simulink library "my_library"  (R2014a)
settings: Solver=ode45  StartTime=0.0  StopTime=10.0  RelTol=1e-3
values from neighbouring files (symbols this model uses):
  D = D~=0    [diffTimeSeries.m]    (also in scenario_visualizer_gui.m = D+diffTimeSeries(scenario.failure.communication.packet_recei)
undefined symbols (not defined in the file or in its folder): cmd_delay, decStep, decStepMax, incStep
libraries: my_library x27, simulink x1
settings Model: Creator=jean  LastModifiedBy=jean

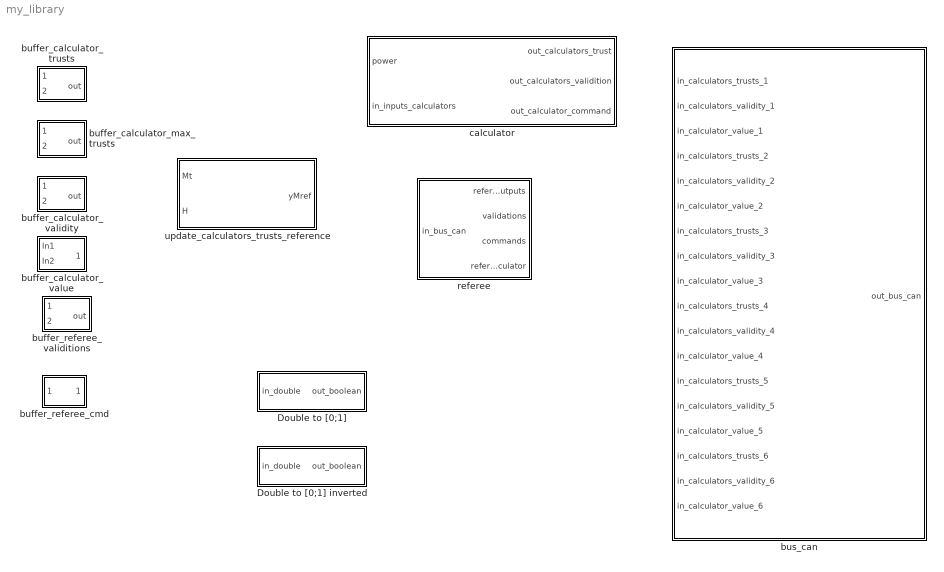
== system my_library ==
  Double to [0;1] : Subsystem
  Double to [0;1] inverted : Subsystem
  buffer_calculator_max_trusts : Subsystem
  buffer_calculator_trusts : Subsystem
  buffer_calculator_validity : Subsystem
  buffer_calculator_value : Subsystem
  buffer_referee_cmd : Subsystem
  buffer_referee_validitions : Subsystem
  bus_can : Subsystem
      mask Display: image('images/network_grid.jpg');
  calculator : Subsystem  mask{id=0}
      mask prompts: id "Component ID"
      mask init:
      | id>=1
      mask Display: image('images/stm32f4_discovery.jpg');
  referee : Subsystem  mask{cmd_delay=4}
      mask prompts: cmd_delay "Command delay"
      mask Display: image('images/984838-brain.jpg');
  update_calculators_trusts_reference : MATLAB Function  TreatAsAtomicUnit=on

== system my_library/Double to [0;1] ==
  in_double : Inport
  Constant : Constant  Value=0
  Constant1 : Constant
  Switch : Switch  Threshold=0.5
  out_boolean : Outport
  wires:
  Constant/1 -> Switch/3
  Constant1/1 -> Switch/1
  Switch/1 -> out_boolean/1
  in_double/1 -> Switch/2

== system my_library/Double to [0;1] inverted ==
  in_double : Inport
  Constant : Constant
  Constant1 : Constant  Value=0
  Switch : Switch  Threshold=0.5
  out_boolean : Outport
  wires:
  in_double/1 -> Switch/2
  Switch/1 -> out_boolean/1
  Constant1/1 -> Switch/1
  Constant/1 -> Switch/3

== system my_library/buffer_calculator_max_trusts ==
  input : Inport
  reset : Inport  Port=2
  Delay18 : Delay  DelayLength=1  InitialCondition=ones(1,9,'double')  ExternalReset=Level hold
      settings: InputPortMap=u0,r5
  Reshape12 : Reshape  OutputDimensionality=Row vector (2-D)  OutputDimensions=[6,6]
  out : Outport
  wires:
  Delay18/1 -> Reshape12/1
  input/1 -> Delay18/1
  Reshape12/1 -> out/1
  reset/1 -> Delay18/2

== system my_library/buffer_calculator_trusts ==
  input : Inport
  reset : Inport  Port=2
  Reshape : Reshape  OutputDimensionality=Row vector (2-D)  OutputDimensions=[6,6]
  calculator_buffer_trusts : Delay  DelayLength=1  InitialCondition=ones(1,6,'double')  ExternalReset=Level hold
      settings: InputPortMap=u0,r5
  out : Outport
  wires:
  reset/1 -> calculator_buffer_trusts/2
  calculator_buffer_trusts/1 -> Reshape/1
  input/1 -> calculator_buffer_trusts/1
  Reshape/1 -> out/1

== system my_library/buffer_calculator_validity ==
  input : Inport
  reset : Inport  Port=2
  Delay6 : Delay  DelayLength=1  InitialCondition=cast(zeros(1,6),'int8')  ExternalReset=Level hold
      settings: InputPortMap=u0,r5
  Reshape6 : Reshape  OutputDimensionality=Row vector (2-D)  OutputDimensions=[6,6]
  out : Outport
  wires:
  input/1 -> Delay6/1
  Reshape6/1 -> out/1
  Delay6/1 -> Reshape6/1
  reset/1 -> Delay6/2

== system my_library/buffer_calculator_value ==
  In1 : Inport
  In2 : Inport  Port=2
  Delay : Delay  DelayLength=1  ExternalReset=Level hold
      settings: InputPortMap=u0,r5
  Out1 : Outport
  wires:
  Delay/1 -> Out1/1
  In1/1 -> Delay/1
  In2/1 -> Delay/2

== system my_library/buffer_referee_cmd ==
  In1 : Inport
  calculators_validity_6 : Delay  DelayLength=cmd_delay  InitialCondition=0
  Out1 : Outport
  wires:
  In1/1 -> calculators_validity_6/1
  calculators_validity_6/1 -> Out1/1

== system my_library/buffer_referee_validitions ==
  input : Inport
  reset : Inport  Port=2
  Delay6 : Delay  DelayLength=cmd_delay-1  InitialCondition=0  ExternalReset=Level hold
      settings: InputPortMap=u0,r5
  Reshape6 : Reshape  OutputDimensionality=Row vector (2-D)  OutputDimensions=[6,6]
  out : Outport
  wires:
  input/1 -> Delay6/1
  Reshape6/1 -> out/1
  Delay6/1 -> Reshape6/1
  reset/1 -> Delay6/2

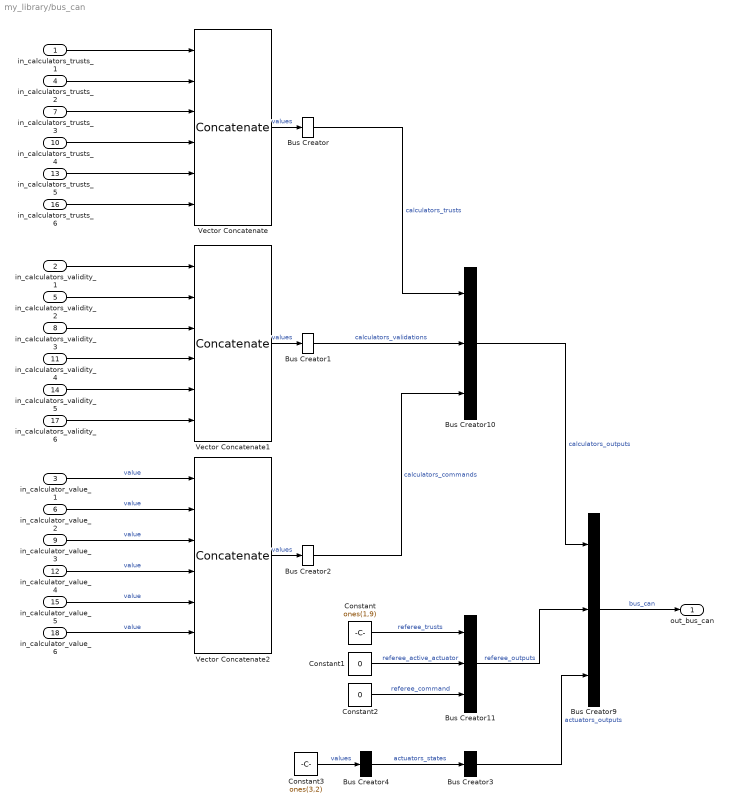
== system my_library/bus_can ==
  in_calculators_trusts_1 : Inport
  in_calculators_validity_1 : Inport  Port=2
  in_calculator_value_1 : Inport  Port=3  OutDataTypeStr=double  PortDimensions=1
  in_calculators_trusts_2 : Inport  Port=4
  in_calculators_validity_2 : Inport  Port=5
  in_calculator_value_2 : Inport  Port=6  OutDataTypeStr=double  PortDimensions=1
  in_calculators_trusts_3 : Inport  Port=7
  in_calculators_validity_3 : Inport  Port=8
  in_calculator_value_3 : Inport  Port=9  OutDataTypeStr=double  PortDimensions=1
  in_calculators_trusts_4 : Inport  Port=10
  in_calculators_validity_4 : Inport  Port=11
  in_calculator_value_4 : Inport  Port=12  OutDataTypeStr=double  PortDimensions=1
  in_calculators_trusts_5 : Inport  Port=13
  in_calculators_validity_5 : Inport  Port=14
  in_calculator_value_5 : Inport  Port=15  OutDataTypeStr=double  PortDimensions=1
  in_calculators_trusts_6 : Inport  Port=16
  in_calculators_validity_6 : Inport  Port=17
  in_calculator_value_6 : Inport  Port=18  OutDataTypeStr=double  PortDimensions=1
  Bus Creator : BusCreator  Inputs=1  OutDataTypeStr=Bus: bus_calculators_trusts
  Bus Creator1 : BusCreator  Inputs=1  OutDataTypeStr=Bus: bus_calculators_validations
  Bus Creator10 : BusCreator  Inputs=3  OutDataTypeStr=Bus: bus_calculators_outputs
  Bus Creator11 : BusCreator  Inputs=3  OutDataTypeStr=Bus: bus_referee_outputs
  Bus Creator2 : BusCreator  Inputs=1  OutDataTypeStr=Bus: bus_calculators_commands
  Bus Creator3 : BusCreator  Inputs=1  OutDataTypeStr=Bus: bus_actuators_outputs
  Bus Creator4 : BusCreator  Inputs=1  OutDataTypeStr=Bus: bus_actuators_states
  Bus Creator9 : BusCreator  Inputs=3  OutDataTypeStr=Bus: bus_can
  Constant : Constant  Value=ones(1,9)
  Constant1 : Constant  Value=0
  Constant2 : Constant  Value=0
  Constant3 : Constant  Value=ones(3,2)  VectorParams1D=off
  Vector Concatenate : Concatenate  NumInputs=6  Mode=Multidimensional array
  Vector Concatenate1 : Concatenate  NumInputs=6  Mode=Multidimensional array
  Vector Concatenate2 : Concatenate  NumInputs=6  Mode=Multidimensional array
  out_bus_can : Outport  OutDataTypeStr=Bus: bus_can
  wires:
  Vector Concatenate/1 -> Bus Creator/1  "values"
  Vector Concatenate1/1 -> Bus Creator1/1  "values"
  Vector Concatenate2/1 -> Bus Creator2/1  "values"
  in_calculators_trusts_4/1 -> Vector Concatenate/4
  in_calculators_trusts_1/1 -> Vector Concatenate/1
  in_calculators_trusts_5/1 -> Vector Concatenate/5
  in_calculators_trusts_3/1 -> Vector Concatenate/3
  in_calculators_trusts_2/1 -> Vector Concatenate/2
  in_calculators_trusts_6/1 -> Vector Concatenate/6
  in_calculators_validity_4/1 -> Vector Concatenate1/4
  in_calculators_validity_1/1 -> Vector Concatenate1/1
  in_calculators_validity_5/1 -> Vector Concatenate1/5
  in_calculators_validity_6/1 -> Vector Concatenate1/6
  in_calculators_validity_3/1 -> Vector Concatenate1/3
  in_calculators_validity_2/1 -> Vector Concatenate1/2
  in_calculator_value_6/1 -> Vector Concatenate2/6  "value"
  in_calculator_value_1/1 -> Vector Concatenate2/1  "value"
  in_calculator_value_3/1 -> Vector Concatenate2/3  "value"
  in_calculator_value_2/1 -> Vector Concatenate2/2  "value"
  in_calculator_value_4/1 -> Vector Concatenate2/4  "value"
  in_calculator_value_5/1 -> Vector Concatenate2/5  "value"
  Bus Creator9/1 -> out_bus_can/1  "bus_can"
  Bus Creator10/1 -> Bus Creator9/1  "calculators_outputs"
  Bus Creator/1 -> Bus Creator10/1  "calculators_trusts"
  Bus Creator1/1 -> Bus Creator10/2  "calculators_validations"
  Bus Creator2/1 -> Bus Creator10/3  "calculators_commands"
  Bus Creator11/1 -> Bus Creator9/2  "referee_outputs"
  Bus Creator3/1 -> Bus Creator9/3  "actuators_outputs"
  Constant/1 -> Bus Creator11/1  "referee_trusts"
  Constant1/1 -> Bus Creator11/2  "referee_active_actuator"
  Constant2/1 -> Bus Creator11/3  "referee_command"
  Bus Creator4/1 -> Bus Creator3/1  "actuators_states"
  Constant3/1 -> Bus Creator4/1  "values"

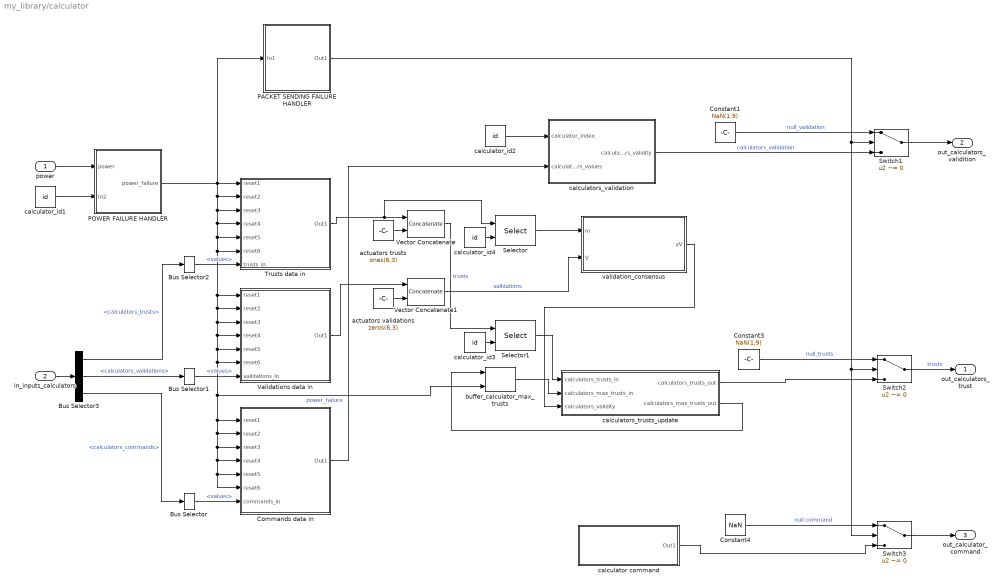
== system my_library/calculator ==
  power : Inport  OutMin=0  OutMax=1  PortDimensions=1
  in_inputs_calculators : Inport  Port=2  OutDataTypeStr=Bus: bus_can
  Bus Selector : BusSelector  OutputSignals=values
  Bus Selector1 : BusSelector  OutputSignals=values
  Bus Selector2 : BusSelector  OutputSignals=values
  Bus Selector3 : BusSelector  OutputSignals=calculators_outputs.calculators_trusts,calculators_outputs.calculators_validations,calculators_outputs.calculators_commands
  Commands data in : Subsystem
  Constant1 : Constant  Value=NaN(1,9)  VectorParams1D=off
  Constant3 : Constant  Value=NaN(1,9)  VectorParams1D=off
  Constant4 : Constant  Value=NaN  VectorParams1D=off
  PACKET SENDING FAILURE HANDLER : Subsystem
  POWER FAILURE HANDLER : Subsystem
      mask Display: image('images/electricity_failure.jpg');
  Selector : Selector  NumberOfDimensions=2  InputPortWidth=6  IndexOptions=Index vector (port),Select all  Indices=[1 3],1  OutputSizes=1,1
  Selector1 : Selector  NumberOfDimensions=2  InputPortWidth=6  IndexOptions=Index vector (port),Select all  Indices=[1 3],1  OutputSizes=1,1
  Switch1 : Switch  Criteria=u2 ~= 0
  Switch2 : Switch  Criteria=u2 ~= 0
  Switch3 : Switch  Criteria=u2 ~= 0
  Trusts data in : Subsystem
  Validations data in : Subsystem
  Vector Concatenate : Concatenate  Mode=Multidimensional array  ConcatenateDimension=2
  Vector Concatenate1 : Concatenate  Mode=Multidimensional array  ConcatenateDimension=2
  actuators trusts : Constant  Value=ones(6,3)  VectorParams1D=off
  actuators validations : Constant  Value=zeros(6,3)  VectorParams1D=off
  buffer_calculator_max_trusts : my_library/buffer_calculator_max_trusts
  calculator command : Subsystem
  calculator_id{1..4} (4 alike) : Constant  Value=id  OutDataTypeStr=uint8
  calculators_trusts_update : Subsystem
  calculators_validation : Subsystem
  validation_consensus : MATLAB Function  TreatAsAtomicUnit=on
  out_calculators_trust : Outport
  out_calculators_validition : Outport  Port=2
  out_calculator_command : Outport  Port=3  OutDataTypeStr=double  PortDimensions=1
  wires:
  calculator_id1/1 -> POWER FAILURE HANDLER/2(In2)
  in_inputs_calculators/1 -> Bus Selector3/1
  validation_consensus/1(yV) -> calculators_trusts_update/3(calculators_validity)
  calculators_trusts_update/1(calculators_trusts_out) -> Switch2/3
  Selector/1 -> validation_consensus/1(m)
  calculators_trusts_update/2(calculators_max_trusts_out) -> buffer_calculator_max_trusts/1
  buffer_calculator_max_trusts/1 -> calculators_trusts_update/2(calculators_max_trusts_in)
  Switch1/1 -> out_calculators_validition/1
  calculators_validation/1(calculators_validity) -> Switch1/3  "calculators_validation"
  Constant1/1 -> Switch1/1  "null_validation"
  Switch2/1 -> out_calculators_trust/1  "trusts"
  Constant3/1 -> Switch2/1  "null_trusts"
  Switch3/1 -> out_calculator_command/1
  Constant4/1 -> Switch3/1  "null command"
  POWER FAILURE HANDLER/1(power_failure) -> buffer_calculator_max_trusts/2, Commands data in/6(reset6), Commands data in/5(reset5), Commands data in/4(reset4), Commands data in/3(reset3), Commands data in/2(reset2), Commands data in/1(reset1), Validations data in/6(reset6), Validations data in/5(reset5), Validations data in/4(reset4), Validations data in/3(reset3), Validations data in/2(reset2), Validations data in/1(reset1), Trusts data in/6(reset6), Trusts data in/5(reset5), Trusts data in/4(reset4), Trusts data in/3(reset3), Trusts data in/2(reset2), PACKET SENDING FAILURE HANDLER/1(In1), Trusts data in/1(reset1)  "power_failure"
  power/1 -> POWER FAILURE HANDLER/1(power)
  Bus Selector3/1 -> Bus Selector2/1  "<calculators_trusts>"
  Trusts data in/1(Out1) -> Selector/1, Vector Concatenate/1
  Bus Selector3/2 -> Bus Selector1/1  "<calculators_validations>"
  Bus Selector/1 -> Commands data in/7(commands_in)  "<values>"
  Commands data in/1(Out1) -> calculators_validation/2(calculators_values)
  calculator_id2/1 -> calculators_validation/1(calculator_index)
  actuators trusts/1 -> Vector Concatenate/2
  calculator_id4/1 -> Selector/2
  actuators validations/1 -> Vector Concatenate1/2
  Validations data in/1(Out1) -> Vector Concatenate1/1
  Vector Concatenate1/1 -> validation_consensus/2(V)  "validations"
  calculator command/1(Out1) -> Switch3/3
  calculator_id3/1 -> Selector1/2
  Vector Concatenate/1 -> Selector1/1  "trusts"
  Selector1/1 -> calculators_trusts_update/1(calculators_trusts_in)
  Bus Selector3/3 -> Bus Selector/1  "<calculators_commands>"
  Bus Selector1/1 -> Validations data in/7(validations_in)  "<values>"
  Bus Selector2/1 -> Trusts data in/7(trusts_in)  "<values>"
  PACKET SENDING FAILURE HANDLER/1(Out1) -> Switch3/2, Switch2/2, Switch1/2

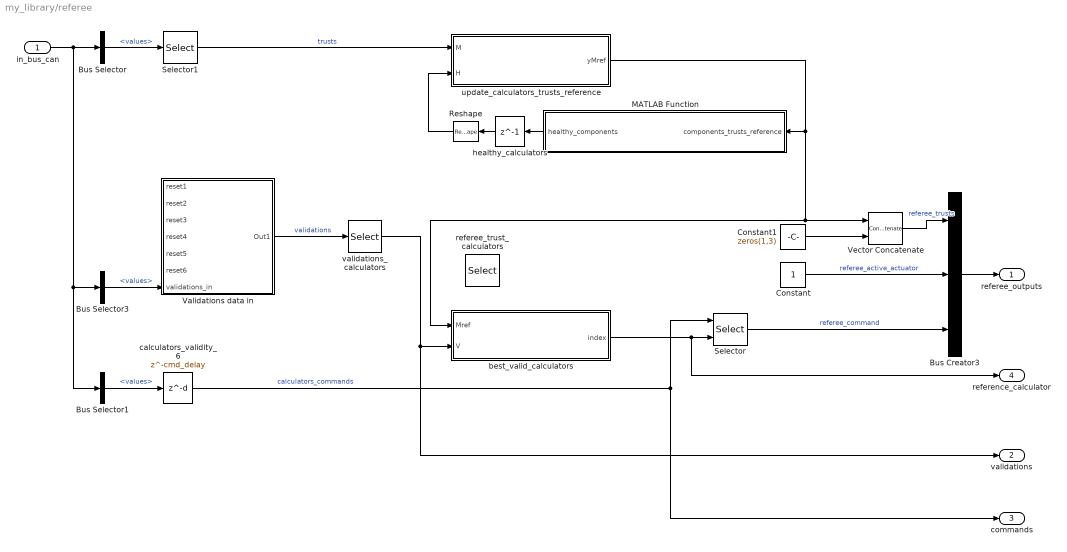
== system my_library/referee ==
  in_bus_can : Inport  OutDataTypeStr=Bus: bus_can
  Bus Creator3 : BusCreator  Inputs=3  OutDataTypeStr=Bus: bus_referee_outputs
  Bus Selector : BusSelector  OutputSignals=calculators_outputs.calculators_trusts.values
  Bus Selector1 : BusSelector  OutputSignals=calculators_outputs.calculators_commands.values
  Bus Selector3 : BusSelector  OutputSignals=calculators_outputs.calculators_validations.values
  Constant : Constant
  Constant1 : Constant  Value=zeros(1,3)  VectorParams1D=off
  MATLAB Function : MATLAB Function  TreatAsAtomicUnit=on
  Reshape : Reshape  OutputDimensionality=Row vector (2-D)
  Selector : Selector  InputPortWidth=6  IndexOptions=Index vector (port)
  Selector1 : Selector  NumberOfDimensions=2  InputPortWidth=3  IndexOptions=Select all,Index vector (dialog)  Indices=,[1:6]  OutputSizes=1,1
  Validations data in : Subsystem
  Vector Concatenate : Concatenate  Mode=Multidimensional array  ConcatenateDimension=2
  best_valid_calculators : MATLAB Function  TreatAsAtomicUnit=on
  calculators_validity_6 : Delay  DelayLength=cmd_delay  InitialCondition=0
  healthy_calculators : Delay  DelayLength=1  InitialCondition=ones(1,6,'uint8')
  referee_trust_calculators : Selector  InputPortWidth=9  Indices=[1:6]
  update_calculators_trusts_reference : MATLAB Function  TreatAsAtomicUnit=on
  validations_calculators : Selector  NumberOfDimensions=2  InputPortWidth=3  IndexOptions=Select all,Index vector (dialog)  Indices=,[1:6]  OutputSizes=1,1
  referee_outputs : Outport  OutDataTypeStr=Bus: bus_referee_outputs
  validations : Outport  Port=2
  commands : Outport  Port=3
  reference_calculator : Outport  Port=4
  wires:
  update_calculators_trusts_reference/1(yMref) -> Vector Concatenate/1, best_valid_calculators/1(Mref), MATLAB Function/1(components_trusts_reference)
  Validations data in/1(Out1) -> validations_calculators/1  "validations"
  calculators_validity_6/1 -> commands/1, Selector/1  "calculators_commands"
  best_valid_calculators/1(index) -> reference_calculator/1, Selector/2
  healthy_calculators/1 -> Reshape/1
  Reshape/1 -> update_calculators_trusts_reference/2(H)
  MATLAB Function/1(healthy_components) -> healthy_calculators/1
  Selector1/1 -> update_calculators_trusts_reference/1(M)  "trusts"
  in_bus_can/1 -> Bus Selector/1, Bus Selector1/1, Bus Selector3/1
  Bus Selector/1 -> Selector1/1  "<values>"
  Bus Selector3/1 -> Validations data in/7(validations_in)  "<values>"
  validations_calculators/1 -> best_valid_calculators/2(V), validations/1
  Bus Selector1/1 -> calculators_validity_6/1  "<values>"
  Constant/1 -> Bus Creator3/2  "referee_active_actuator"
  Selector/1 -> Bus Creator3/3  "referee_command"
  Bus Creator3/1 -> referee_outputs/1
  Vector Concatenate/1 -> Bus Creator3/1  "referee_trusts"
  Constant1/1 -> Vector Concatenate/2

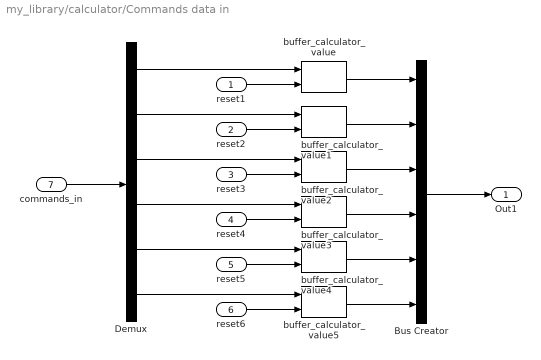
== system my_library/calculator/Commands data in ==
  reset1 : Inport
  reset2 : Inport  Port=2
  reset3 : Inport  Port=3
  reset4 : Inport  Port=4
  reset5 : Inport  Port=5
  reset6 : Inport  Port=6
  commands_in : Inport  Port=7
  Bus Creator : BusCreator  Inputs=6
  Demux : Demux  Outputs=6
  buffer_calculator_value{,1..5} (6 alike) : my_library/buffer_calculator_value
  Out1 : Outport
  wires:
  buffer_calculator_value/1 -> Bus Creator/1
  Bus Creator/1 -> Out1/1
  commands_in/1 -> Demux/1
  buffer_calculator_value5/1 -> Bus Creator/6
  buffer_calculator_value1/1 -> Bus Creator/2
  buffer_calculator_value4/1 -> Bus Creator/5
  buffer_calculator_value3/1 -> Bus Creator/4
  buffer_calculator_value2/1 -> Bus Creator/3
  Demux/4 -> buffer_calculator_value3/1
  Demux/6 -> buffer_calculator_value5/1
  Demux/3 -> buffer_calculator_value2/1
  Demux/1 -> buffer_calculator_value/1
  Demux/5 -> buffer_calculator_value4/1
  Demux/2 -> buffer_calculator_value1/1
  reset3/1 -> buffer_calculator_value2/2
  reset2/1 -> buffer_calculator_value1/2
  reset6/1 -> buffer_calculator_value5/2
  reset1/1 -> buffer_calculator_value/2
  reset5/1 -> buffer_calculator_value4/2
  reset4/1 -> buffer_calculator_value3/2

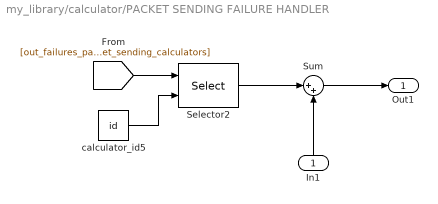
== system my_library/calculator/PACKET SENDING FAILURE HANDLER ==
  In1 : Inport
  Selector2 : Selector  InputPortWidth=6  IndexOptions=Index vector (port)  Indices=[1 3]
  Sum : Sum  Inputs=|++
  calculator_id5 : Constant  Value=id  OutDataTypeStr=uint8
  Out1 : Outport
  wires:
  [out_failures_packet_sending_calculators] -> Selector2/1
  Selector2/1 -> Sum/1
  calculator_id5/1 -> Selector2/2
  In1/1 -> Sum/2
  Sum/1 -> Out1/1

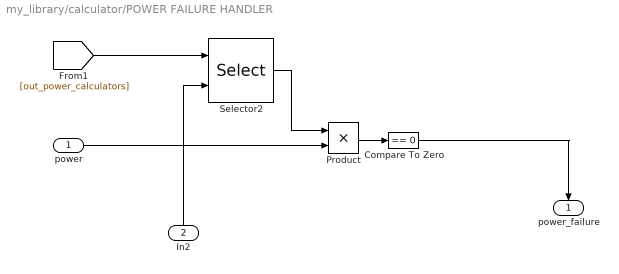
== system my_library/calculator/POWER FAILURE HANDLER ==
  power : Inport  OutMin=0  OutMax=1  PortDimensions=1
  In2 : Inport  Port=2
  Compare To Zero : simulink/Logic and Bit Operations/Compare To Zero  relop===  OutDataTypeStr=boolean
  Product : Product
  Selector2 : Selector  InputPortWidth=6  IndexOptions=Index vector (port)  Indices=[1 3]
  power_failure : Outport
  wires:
  Selector2/1 -> Product/1
  [out_power_calculators] -> Selector2/1
  Product/1 -> Compare To Zero/1
  Compare To Zero/1 -> power_failure/1
  power/1 -> Product/2
  In2/1 -> Selector2/2

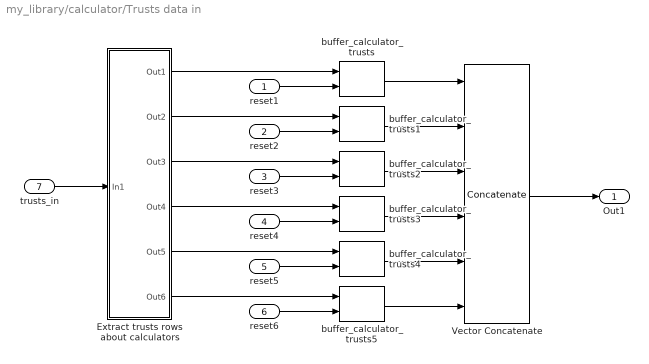
== system my_library/calculator/Trusts data in ==
  reset1 : Inport
  reset2 : Inport  Port=2
  reset3 : Inport  Port=3
  reset4 : Inport  Port=4
  reset5 : Inport  Port=5
  reset6 : Inport  Port=6
  trusts_in : Inport  Port=7
  Extract trusts rows about calculators : Subsystem
  Vector Concatenate : Concatenate  NumInputs=6  Mode=Multidimensional array
  buffer_calculator_trusts{,1..5} (6 alike) : my_library/buffer_calculator_trusts
  Out1 : Outport
  wires:
  buffer_calculator_trusts1/1 -> Vector Concatenate/2
  Vector Concatenate/1 -> Out1/1
  buffer_calculator_trusts3/1 -> Vector Concatenate/4
  buffer_calculator_trusts4/1 -> Vector Concatenate/5
  buffer_calculator_trusts5/1 -> Vector Concatenate/6
  buffer_calculator_trusts/1 -> Vector Concatenate/1
  buffer_calculator_trusts2/1 -> Vector Concatenate/3
  Extract trusts rows about calculators/5(Out5) -> buffer_calculator_trusts4/1
  Extract trusts rows about calculators/6(Out6) -> buffer_calculator_trusts5/1
  trusts_in/1 -> Extract trusts rows about calculators/1(In1)
  Extract trusts rows about calculators/1(Out1) -> buffer_calculator_trusts/1
  Extract trusts rows about calculators/2(Out2) -> buffer_calculator_trusts1/1
  Extract trusts rows about calculators/3(Out3) -> buffer_calculator_trusts2/1
  Extract trusts rows about calculators/4(Out4) -> buffer_calculator_trusts3/1
  reset1/1 -> buffer_calculator_trusts/2
  reset3/1 -> buffer_calculator_trusts2/2
  reset2/1 -> buffer_calculator_trusts1/2
  reset6/1 -> buffer_calculator_trusts5/2
  reset5/1 -> buffer_calculator_trusts4/2
  reset4/1 -> buffer_calculator_trusts3/2

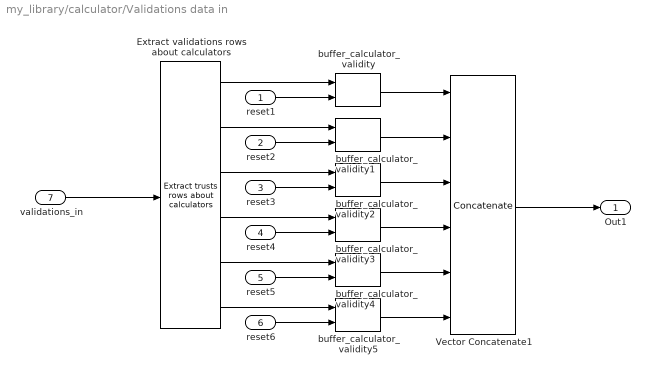
== system my_library/calculator/Validations data in ==
  reset1 : Inport
  reset2 : Inport  Port=2
  reset3 : Inport  Port=3
  reset4 : Inport  Port=4
  reset5 : Inport  Port=5
  reset6 : Inport  Port=6
  validations_in : Inport  Port=7
  Extract validations rows about calculators : my_library/calculator/Trusts data in/Extract trusts rows about calculators
  Vector Concatenate1 : Concatenate  NumInputs=6  Mode=Multidimensional array
  buffer_calculator_validity{,1..5} (6 alike) : my_library/buffer_calculator_validity
  Out1 : Outport
  wires:
  reset3/1 -> buffer_calculator_validity2/2
  reset2/1 -> buffer_calculator_validity1/2
  reset6/1 -> buffer_calculator_validity5/2
  reset1/1 -> buffer_calculator_validity/2
  reset5/1 -> buffer_calculator_validity4/2
  reset4/1 -> buffer_calculator_validity3/2
  Vector Concatenate1/1 -> Out1/1
  buffer_calculator_validity/1 -> Vector Concatenate1/1
  buffer_calculator_validity5/1 -> Vector Concatenate1/6
  buffer_calculator_validity3/1 -> Vector Concatenate1/4
  validations_in/1 -> Extract validations rows about calculators/1
  buffer_calculator_validity4/1 -> Vector Concatenate1/5
  buffer_calculator_validity1/1 -> Vector Concatenate1/2
  buffer_calculator_validity2/1 -> Vector Concatenate1/3
  Extract validations rows about calculators/2 -> buffer_calculator_validity1/1
  Extract validations rows about calculators/3 -> buffer_calculator_validity2/1
  Extract validations rows about calculators/4 -> buffer_calculator_validity3/1
  Extract validations rows about calculators/5 -> buffer_calculator_validity4/1
  Extract validations rows about calculators/1 -> buffer_calculator_validity/1
  Extract validations rows about calculators/6 -> buffer_calculator_validity5/1

== system my_library/calculator/calculator command ==
  Selector1 : Selector  InputPortWidth=6  IndexOptions=Index vector (port)  Indices=[1 3]
  calculator_id3 : Constant  Value=id  OutDataTypeStr=uint8
  Out1 : Outport
  wires:
  [out_calculators] -> Selector1/1  "calculators commands"
  Selector1/1 -> Out1/1  "calculator_command"
  calculator_id3/1 -> Selector1/2

== system my_library/calculator/calculators_trusts_update ==
  calculators_trusts_in : Inport
  calculators_max_trusts_in : Inport  Port=2
  calculators_validity : Inport  Port=3
  MATLAB Function7 : MATLAB Function  TreatAsAtomicUnit=on
  calculators_trusts_out : Outport
  calculators_max_trusts_out : Outport  Port=2
  wires:
  calculators_trusts_in/1 -> MATLAB Function7/1(M)
  calculators_max_trusts_in/1 -> MATLAB Function7/2(Mmax)
  calculators_validity/1 -> MATLAB Function7/3(V)
  MATLAB Function7/1(yM) -> calculators_trusts_out/1  "trusts"
  MATLAB Function7/2(yMmax) -> calculators_max_trusts_out/1  "trusts"

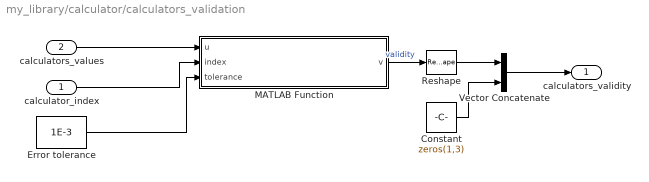
== system my_library/calculator/calculators_validation ==
  calculator_index : Inport  OutDataTypeStr=uint8  PortDimensions=1
  calculators_values : Inport  Port=2  OutDataTypeStr=double
  Constant : Constant  Value=zeros(1,3)  VectorParams1D=off
  Error tolerance : Constant  Value=1E-3
  MATLAB Function : MATLAB Function  TreatAsAtomicUnit=on
  Reshape : Reshape  OutputDimensionality=Row vector (2-D)
  Vector Concatenate : Concatenate
  calculators_validity : Outport
  wires:
  Error tolerance/1 -> MATLAB Function/3(tolerance)
  calculators_values/1 -> MATLAB Function/1(u)
  MATLAB Function/1(v) -> Reshape/1  "validity"
  calculator_index/1 -> MATLAB Function/2(index)
  Reshape/1 -> Vector Concatenate/1
  Constant/1 -> Vector Concatenate/2
  Vector Concatenate/1 -> calculators_validity/1

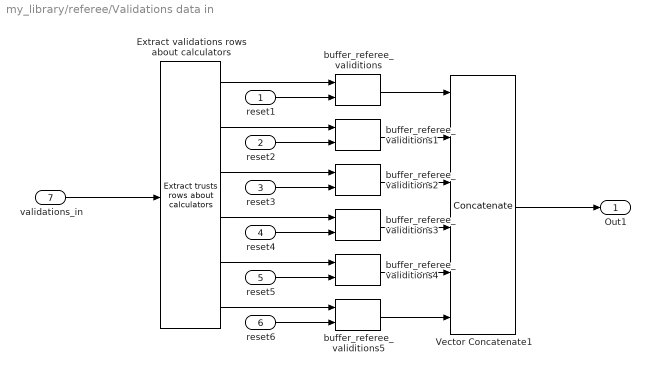
== system my_library/referee/Validations data in ==
  reset1 : Inport
  reset2 : Inport  Port=2
  reset3 : Inport  Port=3
  reset4 : Inport  Port=4
  reset5 : Inport  Port=5
  reset6 : Inport  Port=6
  validations_in : Inport  Port=7
  Extract validations rows about calculators : my_library/calculator/Trusts data in/Extract trusts rows about calculators
  Vector Concatenate1 : Concatenate  NumInputs=6  Mode=Multidimensional array
  buffer_referee_validitions{,1..5} (6 alike) : my_library/buffer_referee_validitions
  Out1 : Outport
  wires:
  Extract validations rows about calculators/6 -> buffer_referee_validitions5/1
  Extract validations rows about calculators/1 -> buffer_referee_validitions/1
  Extract validations rows about calculators/5 -> buffer_referee_validitions4/1
  Extract validations rows about calculators/4 -> buffer_referee_validitions3/1
  Extract validations rows about calculators/3 -> buffer_referee_validitions2/1
  Extract validations rows about calculators/2 -> buffer_referee_validitions1/1
  buffer_referee_validitions2/1 -> Vector Concatenate1/3
  buffer_referee_validitions1/1 -> Vector Concatenate1/2
  buffer_referee_validitions4/1 -> Vector Concatenate1/5
  validations_in/1 -> Extract validations rows about calculators/1
  buffer_referee_validitions3/1 -> Vector Concatenate1/4
  buffer_referee_validitions5/1 -> Vector Concatenate1/6
  buffer_referee_validitions/1 -> Vector Concatenate1/1
  Vector Concatenate1/1 -> Out1/1
  reset4/1 -> buffer_referee_validitions3/2
  reset5/1 -> buffer_referee_validitions4/2
  reset1/1 -> buffer_referee_validitions/2
  reset6/1 -> buffer_referee_validitions5/2
  reset2/1 -> buffer_referee_validitions1/2
  reset3/1 -> buffer_referee_validitions2/2

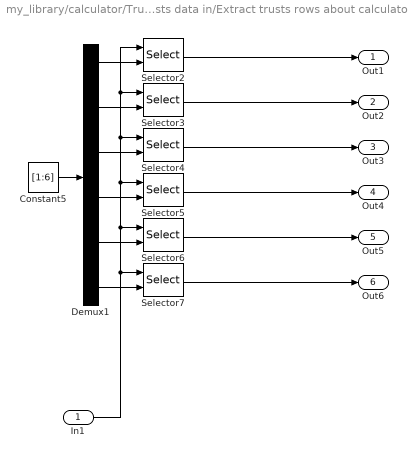
== system my_library/calculator/Trusts data in/Extract trusts rows about calculators ==
  In1 : Inport
  Constant5 : Constant  Value=[1:6]
  Demux1 : Demux  Outputs=6
  Selector{2..7} (6 alike) : Selector  NumberOfDimensions=2  InputPortWidth=3  IndexOptions=Index vector (port),Index vector (dialog)  Indices=1,[1:6]  OutputSizes=1,1
  Out1 : Outport
  Out2 : Outport  Port=2
  Out3 : Outport  Port=3
  Out4 : Outport  Port=4
  Out5 : Outport  Port=5
  Out6 : Outport  Port=6
  wires:
  Demux1/2 -> Selector3/2
  Demux1/3 -> Selector4/2
  In1/1 -> Selector7/1, Selector6/1, Selector5/1, Selector4/1, Selector3/1, Selector2/1
  Selector2/1 -> Out1/1
  Selector6/1 -> Out5/1
  Selector3/1 -> Out2/1
  Selector4/1 -> Out3/1
  Selector5/1 -> Out4/1
  Demux1/6 -> Selector7/2
  Selector7/1 -> Out6/1
  Constant5/1 -> Demux1/1
  Demux1/1 -> Selector2/2
  Demux1/5 -> Selector6/2
  Demux1/4 -> Selector5/2

== matlab function my_library/calculator/validation_consensus ==
  data: m input; yV output; V input
function yV = validation_consensus(m,V)

m(isnan(m))=0;
V(isnan(V))=0;

yV=(m*V>=0).*2-1;

assert(sum(isnan(yV))==0);

== matlab function my_library/calculator/calculators_validation/MATLAB Function ==
  data: u input; index input; v output; tolerance input
function v = validation_data_all(u, index, tolerance)

%
%u=[1 2 1.1 NaN NaN NaN]';
%index=1;
%tolerance=0.5;

% u est un vecteur ligne de données (ex: mesures de 3 capteurs : [0.1 0.11 0.2])
n = size(u,1);
v=zeros(1,n);

if(isnan(u(index))) v=zeros(1,6);
else
    for i=1:n
        if(isnan(u(i)))
            v(i)=-1;
        else
            v(i)=(abs(u(i)-u(index))>tolerance)*(-2)+1;
        end
    end
end

assert(sum(isnan(v))==0)

== matlab function my_library/referee/MATLAB Function ==
  data: components_trusts_reference input; healthy_components output boolean
function healthy_components = update_healthy_components(components_trusts_reference)
%#codegen

healthy_components = logical(components_trusts_reference>=0.5);

== matlab function my_library/update_calculators_trusts_reference ==
  data: Mt input; yMref output; H input
function yMref  = update_trusts_reference(Mt, H)

M=Mt';
% M = confiance,
% H = population saine
%M=[ones(6,3) zeros(6,1) ones(6,1) zeros(6,1)]
%M=[1.0 1.0 0.9 1.0 0.2 0.1; 1.0 1.0 1.0 1.0 0.2 0.1; 0.9 0.9 1.0 1.0 0.2 0.2; 1.0 0.9 0.8 0.9 0.3 0.2; 0 0 0 0 0.8 0.7; 0 0 0 0 0.8 0.9];
%H=ones(1,6);
if(size(H,1)>size(H,2))
    Ht=H'; % si H vecteur ligne transformé en vecteur colonne
end

n=size(M,1);
alpha=zeros(n,n);

M(isnan(M))=0;

for i=1:n
    G=zeros(1,n);
    G(i)=1;
    alpha(i,:)=((G.*Ht)*M)*(Ht*M*G');
end

yMref=sum(alpha)/max(sum(alpha));

== matlab function my_library/calculator/calculators_trusts_update/MATLAB Function7 ==
  data: M input; yM output; Mmax input; V input; incStep parameter; decStep parameter; yMmax output; decStepMax parameter
function [yM, yMmax] = trust_update(M,Mmax,V,incStep,decStep,decStepMax)
%#codegen

M(isnan(M))=0;
V(isnan(V))=0;

Vpos = V>0; % pas d'erreur
Vpos = cast(Vpos,'double');
Vneg = V<0; % erreur
Vneg = cast(Vneg,'double');

yM1=M+(Mmax.*Vpos*incStep)-(Mmax.*Vneg*decStep); % mise à jour de M
yM2=(yM1.*(yM1<Mmax))+(Mmax.*(yM1>=Mmax)); % valeurs max. < à Mmax
yM=(yM2.*(yM2>=0)); % valeurs min >= 0

deltaM = M-yM; % écart : positif si confiance perdue
yMmax=Mmax-(deltaM.*(deltaM>0).*decStepMax);

assert(sum(isnan(yM))==0);
assert(sum(isnan(yMmax))==0);

== matlab function my_library/referee/best_valid_calculators ==
  data: Mref input; index output; V input
function index = best_valid_component_index(Mref,V)

%%
% M=[1.0 1.0 0.9 1.0 0.2 0.1];
% V=[1 1 -1 -1 -1 1; 1 1 -1 -1 -1 -1; -1 -1 1 -1 -1 1; -1 -1 -1 1 -1 -1; -1 -1 -1 -1 1 1; 1 -1 1 -1 1 1];

Mref(isnan(Mref))=0;
V(isnan(V))=0;

yV=(Mref*V>=0);
[v,index]=max(Mref.*yV);

== matlab function my_library/referee/update_calculators_trusts_reference ==
  data: M input; yMref output; H input
function yMref  = update_trusts_reference(M, H)

% M = confiance,
% H = population saine
%M=[ones(6,3) zeros(6,1) ones(6,1) zeros(6,1)]
%M=[1.0 1.0 0.9 1.0 0.2 0.1; 1.0 1.0 1.0 1.0 0.2 0.1; 0.9 0.9 1.0 1.0 0.2 0.2; 1.0 0.9 0.8 0.9 0.3 0.2; 0 0 0 0 0.8 0.7; 0 0 0 0 0.8 0.9];
%H=ones(1,6);

%M=[1 NaN; 2 3];
%H=[1 1];

n=size(M,1);
alpha=zeros(n,n);

M(isnan(M))=0;

for i=1:n
    G=zeros(1,n);
    G(i)=1;
    alpha(i,:)=((G.*H)*M)*(H*M*G');
end

yMref=sum(alpha)/max(sum(alpha));

if(sum(isnan(yMref))>0)
    for i=1:n
        G=zeros(1,n);
        G(i)=1;
        alpha(i,:)=(G*M)*(ones(1,n)*M*G');
    end

    yMref=sum(alpha)/max(sum(alpha));
end
